simulink model "Design"  (R2023b)
settings: Solver=VariableStepAuto  StartTime=0.0  StopTime=10.0  RelTol=1e-3
libraries: cstblocks x8
settings Model: Creator=randolf  LastModifiedBy=randolf

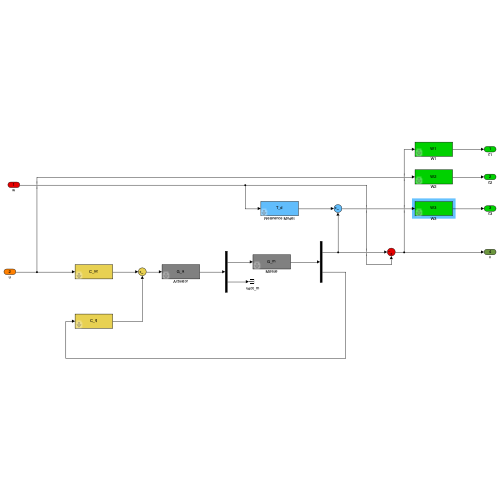
[thumbnail: Simulink's stored preview of the top-level diagram]
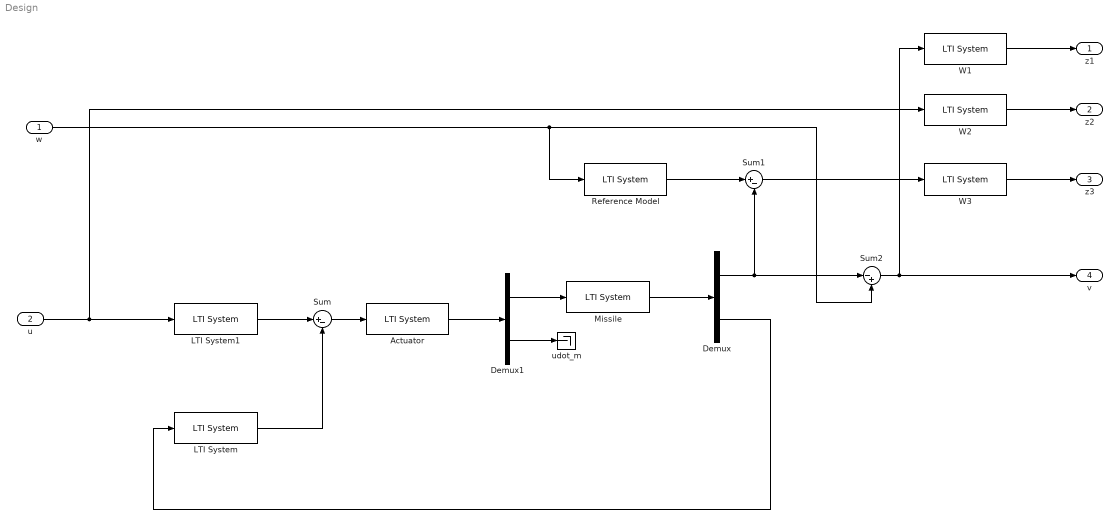
== system Design ==
  w : Inport
  u : Inport  Port=2
  Actuator : cstblocks/LTI System  sys=G_a  IC=[]  PadeOrder=0
  Demux : Demux  Outputs=2
  Demux1 : Demux  Outputs=2
  LTI System : cstblocks/LTI System  sys=C_q  IC=[]  PadeOrder=0
  LTI System1 : cstblocks/LTI System  sys=C_sc  IC=[]  PadeOrder=0
  Missile : cstblocks/LTI System  sys=G_m  IC=[]  PadeOrder=0
  Reference Model : cstblocks/LTI System  sys=T_d  IC=[]  PadeOrder=0
  Sum : Sum  Inputs=|+-
  Sum1 : Sum  Inputs=|+-
  Sum2 : Sum  Inputs=|-+
  W1 : cstblocks/LTI System  sys=W1  IC=[]  PadeOrder=0
  W2 : cstblocks/LTI System  sys=W2  IC=[]  PadeOrder=0
  W3 : cstblocks/LTI System  sys=W3  IC=[]  PadeOrder=0
  udot_m : Terminator
  z1 : Outport
  z2 : Outport  Port=2
  z3 : Outport  Port=3
  v : Outport  Port=4
  wires:
  LTI System1/1 -> Sum/1
  Missile/1 -> Demux/1
  Demux/1 -> Sum2/1, Sum1/2
  LTI System/1 -> Sum/2
  Actuator/1 -> Demux1/1
  Sum/1 -> Actuator/1
  Demux1/1 -> Missile/1
  Demux/2 -> LTI System/1
  Demux1/2 -> udot_m/1
  Reference Model/1 -> Sum1/1
  w/1 -> Reference Model/1, Sum2/2
  u/1 -> W2/1, LTI System1/1
  Sum1/1 -> W3/1
  W1/1 -> z1/1
  W2/1 -> z2/1
  W3/1 -> z3/1
  Sum2/1 -> W1/1, v/1
